simulink model "LQ_with_noise_realistic"  (R2023a)
settings: Solver=ode4  StartTime=0.0  StopTime=10  FixedStep=0.001  RelTol=1e-3
InitFcn:
  | Init_control;
values from neighbouring files (symbols this model uses):
  D = zeros(2,4)    [Init_control.m]
  klq = lqrd(A,B,Q,Rlq,Ts)    [Init_control.m]
  ModelInit_AngEuler = [0.4, 0.2, 0]    [Init_control.m]
  ModelInit_PosE = [0, 0, -100]    [Init_control.m]
  ModelInit_Rads = 557.142    [Init_control.m]
  ModelInit_RateB = [0, 0, 0]    [Init_control.m]
  ModelInit_VelB = [0, 0, 0]    [Init_control.m]
  P = [0.5 0 0 0 ... (first row only)    [Init_control.m]
  R = sqrt(2)/2*[-1 1 ... (first row only)    [Init_control.m]
  Ts = 0.002    [Init_control.m]
undefined symbols (not defined in the file or in its folder): ModelParam_envGravityAcc, ModelParam_motorCr, ModelParam_motorJm, ModelParam_motorT, ModelParam_motorWb, ModelParam_rotorCm, ModelParam_rotorCt, ModelParam_uavCCm, ModelParam_uavCd, ModelParam_uavJ, ModelParam_uavMass, ModelParam_uavR
libraries: simulink x4, sharedutil x2
settings Model: Creator=wsh  LastModifiedBy=matte
settings SolverCC: AlgebraicLoopSolver=TrustRegion
settings DataIOCC: ReturnWorkspaceOutputs=off
settings DebuggingCC: UnconnectedInputMsg=warning  UnconnectedOutputMsg=warning  UnconnectedLineMsg=warning  BusObjectLabelMismatch=error  ArithmeticOperatorsInVariantConditions=warning
settings ModelReferenceCC: EnableRefExpFcnMdlSchedulingChecks=on
settings SFSimCC: SimUseLocalCustomCode=off  CustomCodeUndefinedFunction=UseInterfaceOnly
settings RTWCC: RTWUseLocalCustomCode=off
settings CodeAppCC: StateflowObjectComments=on

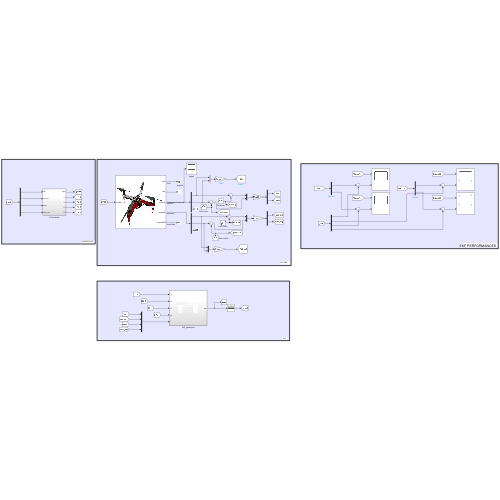
[thumbnail: Simulink's stored preview of the top-level diagram]
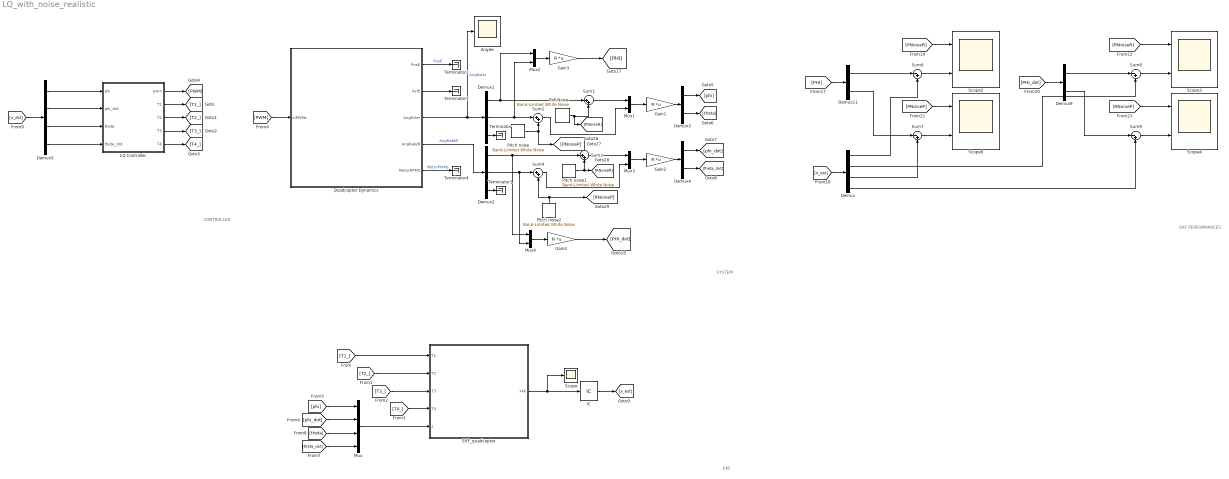
== system LQ_with_noise_realistic ==
  note: SYSTEM
  note: EKF
  note: CONTROLLER
  note: EKF PERFORMANCES
  Angles : Scope
  Demux : Demux
  Demux1 : Demux  Outputs=3
  Demux{3..4,9,11} (4 alike) : Demux  Outputs=2
  Demux2 : Demux  Outputs=3
  Demux5 : Demux
  EKF_quadcopter : Subsystem
  Gain{1..4} (4 alike) : Gain  Gain=R  Multiplication=Matrix(K*u) (u vector)
  IC : InitialCondition  Value=[0;0;0;0]
  LQ Controller : Subsystem
  Mux : Mux
  Mux{1..4} (4 alike) : Mux  Inputs=2
  Pitch noise : simulink/Sources/Band-Limited White Noise  Cov=[1.809123162388460e-08]  Ts=Ts  seed=[23341]
  Pitch noise1 : simulink/Sources/Band-Limited White Noise  Cov=[2.7827391e-06]  Ts=Ts  seed=[23341]
  Pitch noise2 : simulink/Sources/Band-Limited White Noise  Cov=[2.718240466492716e-06]  Ts=Ts  seed=[23341]
  Quadcopter Dynamics : Subsystem
      mask Display: image('./icon/F450.png');
  Roll Noise : simulink/Sources/Band-Limited White Noise  Cov=[1.936548166270313e-08]  Ts=Ts  seed=[23341]
  Scope : Scope
  Scope{2..4,6} (4 alike) : Scope  NumInputPorts=2
  Sum{1..4} (4 alike) : Sum  Inputs=|++
  Sum{6..9} (4 alike) : Sum  Inputs=|-+
  Terminator{,1..4} (5 alike) : Terminator
  wires:
  [x_est] -> Demux5/1
  [PWM] -> Quadcopter Dynamics/1(inPWMs)
  Demux4/2 -> [theta_dot]
  [phi] -> Mux/1
  [theta_dot] -> Mux/4
  Demux5/2 -> LQ Controller/2(phi_dot)
  Demux5/4 -> LQ Controller/4(theta_dot)
  Pitch noise/1 -> [PNoiseP], Sum2/2
  [T4_] -> EKF_quadcopter/4(T4)
  Sum4/1 -> Mux3/2
  IC/1 -> [x_est]
  LQ Controller/3(T2) -> [T2_]
  [theta] -> Mux/3
  Mux1/1 -> Gain1/1
  Demux2/1 -> Mux4/1, Sum3/1
  Sum2/1 -> Mux1/2
  EKF_quadcopter/1(xkk) -> IC/1, Scope/1
  LQ Controller/1(pwm) -> [PWM]
  LQ Controller/4(T3) -> [T3_]
  Demux5/3 -> LQ Controller/3(theta)
  [phi_dot] -> Mux/2
  Sum3/1 -> Mux3/1
  [T3_] -> EKF_quadcopter/3(T3)
  Pitch noise2/1 -> [RNoiseP], Sum4/2
  Demux2/2 -> Mux4/2, Sum4/1
  Demux3/1 -> [phi]
  LQ Controller/2(T1) -> [T1_]
  [T2_] -> EKF_quadcopter/2(T2)
  Quadcopter Dynamics/2(VelE) -> Terminator3/1
  Demux1/2 -> Mux2/2, Sum2/1
  LQ Controller/5(T4) -> [T4_]
  Gain1/1 -> Demux3/1
  Gain2/1 -> Demux4/1
  Roll Noise/1 -> [PNoiseR], Sum1/2
  Quadcopter Dynamics/1(PosE) -> Terminator2/1  "PosE"
  [T1_] -> EKF_quadcopter/1(T1)
  Demux3/2 -> [theta]
  Demux2/3 -> Terminator1/1
  Quadcopter Dynamics/5(MotorRPMS) -> Terminator4/1  "MotorPWMs"
  Demux1/3 -> Terminator/1
  Mux/1 -> EKF_quadcopter/5(z)
  Demux4/1 -> [phi_dot]
  Demux1/1 -> Mux2/1, Sum1/1
  Quadcopter Dynamics/4(AngRateB) -> Demux2/1  "AngRateB"
  Sum1/1 -> Mux1/1
  Demux5/1 -> LQ Controller/1(phi)
  Mux3/1 -> Gain2/1
  Demux/4 -> Sum9/2
  [PHI_dot] -> Demux9/1
  Demux9/1 -> Sum8/1
  Demux9/2 -> Sum9/1
  Demux11/2 -> Sum7/1
  Sum7/1 -> Scope6/2
  Demux/1 -> Sum6/2
  [PHI] -> Demux11/1
  Sum6/1 -> Scope2/2
  Demux11/1 -> Sum6/1
  Demux/3 -> Sum7/2
  Sum8/1 -> Scope3/2
  Sum9/1 -> Scope4/2
  Quadcopter Dynamics/3(AngEuler) -> Demux1/1, Angles/1  "AngEular"
  [x_est] -> Demux/1
  Demux/2 -> Sum8/2
  Pitch noise1/1 -> [RNoiseR], Sum3/2
  [PNoiseR] -> Scope2/1
  [PNoiseP] -> Scope6/1
  [RNoiseR] -> Scope3/1
  [RNoiseP] -> Scope4/1
  Mux2/1 -> Gain3/1
  Gain3/1 -> [PHI]
  Mux4/1 -> Gain4/1
  Gain4/1 -> [PHI_dot]

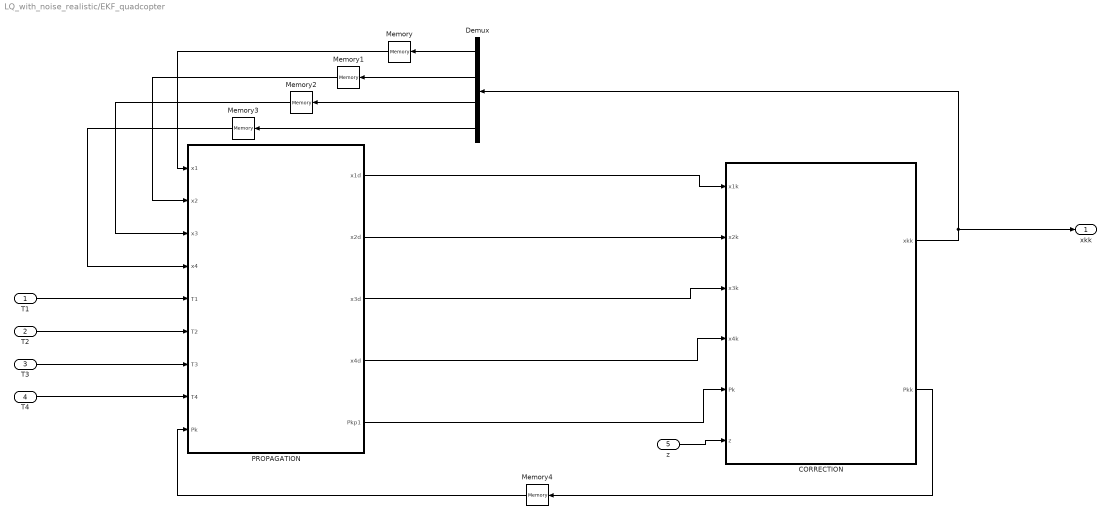
== system LQ_with_noise_realistic/EKF_quadcopter ==
  T1 : Inport
  T2 : Inport  Port=2
  T3 : Inport  Port=3
  T4 : Inport  Port=4
  z : Inport  Port=5
  CORRECTION : MATLAB Function  TreatAsAtomicUnit=on
  Demux : Demux
  Memory{,1..3} (4 alike) : Memory
  Memory4 : Memory  InitialCondition=P
  PROPAGATION : MATLAB Function  TreatAsAtomicUnit=on
  xkk : Outport
  wires:
  PROPAGATION/1(x1d) -> CORRECTION/1(x1k)
  PROPAGATION/2(x2d) -> CORRECTION/2(x2k)
  PROPAGATION/3(x3d) -> CORRECTION/3(x3k)
  PROPAGATION/4(x4d) -> CORRECTION/4(x4k)
  Memory4/1 -> PROPAGATION/9(Pk)
  T1/1 -> PROPAGATION/5(T1)
  T2/1 -> PROPAGATION/6(T2)
  T3/1 -> PROPAGATION/7(T3)
  T4/1 -> PROPAGATION/8(T4)
  PROPAGATION/5(Pkp1) -> CORRECTION/5(Pk)
  CORRECTION/2(Pkk) -> Memory4/1
  z/1 -> CORRECTION/6(z)
  Demux/1 -> Memory/1
  Demux/2 -> Memory1/1
  Demux/3 -> Memory2/1
  Demux/4 -> Memory3/1
  CORRECTION/1(xkk) -> Demux/1, xkk/1
  Memory/1 -> PROPAGATION/1(x1)
  Memory1/1 -> PROPAGATION/2(x2)
  Memory2/1 -> PROPAGATION/3(x3)
  Memory3/1 -> PROPAGATION/4(x4)

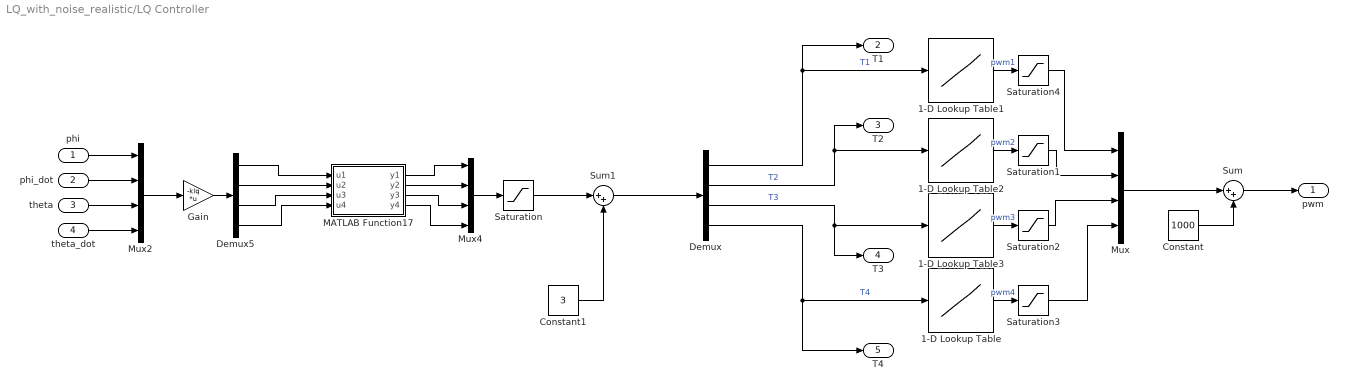
== system LQ_with_noise_realistic/LQ Controller ==
  phi : Inport
  phi_dot : Inport  Port=2
  theta : Inport  Port=3
  theta_dot : Inport  Port=4
  1-D Lookup Table : Lookup_n-D  NumberOfTableDimensions=1  BreakpointsForDimension1=[0;0.06477642396;0.16;0.63;2.44;4.43;6.92;8.77;10.52;11.63;12.03;12.09;12.091;12.092;12.093;12.094;12.095;12.096;12.097;12.098;12.099]  Table=[0;50;100;150;200;250;300;350;400;450;500;550;600;650;700;750;800;850;900;950;1000]  InternalRulePriority=Speed  RndMeth=Simplest
  1-D Lookup Table1 : Lookup_n-D  NumberOfTableDimensions=1  BreakpointsForDimension1=[0;0.02;0.06;0.29;0.73;1.07;1.88;2.91;4;5.06;6.71;7.86;9.41;10.86;11.45;11.82;12.07;12.31;12.52;12.74;12.75]  Table=[0;50;100;150;200;250;300;350;400;450;500;550;600;650;700;750;800;850;900;950;1000]  InternalRulePriority=Speed  RndMeth=Simplest
  1-D Lookup Table2 : Lookup_n-D  NumberOfTableDimensions=1  BreakpointsForDimension1=[0;0.05;0.39;1.67;3.19;5.57;8.07;10.01;10.71;11.06;11.42;11.53;11.55;11.551;11.552;11.553;11.554;11.555;11.556;11.557;11.558]  Table=[0;50;100;150;200;250;300;350;400;450;500;550;600;650;700;750;800;850;900;950;1000]  InternalRulePriority=Speed  RndMeth=Simplest
  1-D Lookup Table3 : Lookup_n-D  NumberOfTableDimensions=1  BreakpointsForDimension1=[0;0.06;0.23;0.89;2.47;3.9;5.86;7.81;9.42;10.12;10.6;11.01;11.34;11.39;11.391;11.392;11.393;11.394;11.395;11.396;11.397]  Table=[0;50;100;150;200;250;300;350;400;450;500;550;600;650;700;750;800;850;900;950;1000]  InternalRulePriority=Speed  RndMeth=Simplest
  Constant : Constant  Value=1000
  Constant1 : Constant  Value=3
  Demux : Demux
  Demux5 : Demux
  Gain : Gain  Gain=-klq  Multiplication=Matrix(K*u) (u vector)
  MATLAB Function17 : MATLAB Function  TreatAsAtomicUnit=on
  Mux : Mux
  Mux2 : Mux
  Mux4 : Mux
  Saturation : Saturate  UpperLimit=10  LowerLimit=0
  Saturation{1..4} (4 alike) : Saturate  UpperLimit=1000  LowerLimit=0
  Sum : Sum  Inputs=|++
  Sum1 : Sum  Inputs=|++
  pwm : Outport
  T1 : Outport  Port=2
  T2 : Outport  Port=3
  T3 : Outport  Port=4
  T4 : Outport  Port=5
  wires:
  Mux4/1 -> Saturation/1
  Mux2/1 -> Gain/1
  theta/1 -> Mux2/3
  1-D Lookup Table1/1 -> Saturation4/1  "pwm1"
  Saturation/1 -> Sum1/1
  Constant1/1 -> Sum1/2
  phi/1 -> Mux2/1
  1-D Lookup Table/1 -> Saturation3/1  "pwm4"
  Saturation4/1 -> Mux/1
  Demux5/2 -> MATLAB Function17/2(u2)
  Demux/1 -> T1/1, 1-D Lookup Table1/1  "T1"
  Gain/1 -> Demux5/1
  Saturation2/1 -> Mux/3
  Demux/4 -> T4/1, 1-D Lookup Table/1  "T4"
  Demux/3 -> T3/1, 1-D Lookup Table3/1  "T3"
  Demux5/4 -> MATLAB Function17/4(u4)
  Saturation1/1 -> Mux/2
  1-D Lookup Table3/1 -> Saturation2/1  "pwm3"
  Demux/2 -> 1-D Lookup Table2/1, T2/1  "T2"
  Sum1/1 -> Demux/1
  1-D Lookup Table2/1 -> Saturation1/1  "pwm2"
  MATLAB Function17/2(y2) -> Mux4/2
  Saturation3/1 -> Mux/4
  Demux5/3 -> MATLAB Function17/3(u3)
  MATLAB Function17/3(y3) -> Mux4/3
  MATLAB Function17/1(y1) -> Mux4/1
  MATLAB Function17/4(y4) -> Mux4/4
  Demux5/1 -> MATLAB Function17/1(u1)
  phi_dot/1 -> Mux2/2
  theta_dot/1 -> Mux2/4
  Sum/1 -> pwm/1
  Mux/1 -> Sum/1
  Constant/1 -> Sum/2

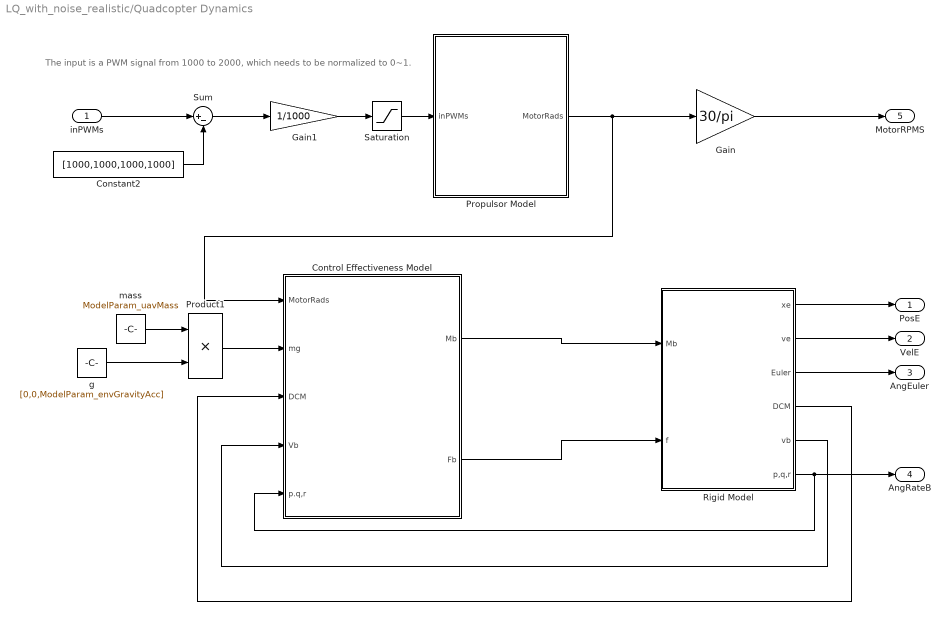
== system LQ_with_noise_realistic/Quadcopter Dynamics ==
  note: The input is a PWM signal from 1000 to 2000,
      | which needs to be normalized to 0~1.
  inPWMs : Inport
  Constant2 : Constant  Value=[1000,1000,1000,1000]
  Control Effectiveness Model : Subsystem
  Gain : Gain  Gain=30/pi
  Gain1 : Gain  Gain=1/1000
  Product1 : Product
  Propulsor Model : Subsystem
  Rigid Model : Subsystem
  Saturation : Saturate  UpperLimit=1  LowerLimit=0
  Sum : Sum  Inputs=|+-
  g : Constant  Value=[0,0,ModelParam_envGravityAcc]
  mass : Constant  Value=ModelParam_uavMass
  PosE : Outport  VectorParamsAs1DForOutWhenUnconnected=off
  VelE : Outport  Port=2  VectorParamsAs1DForOutWhenUnconnected=off
  AngEuler : Outport  Port=3  VectorParamsAs1DForOutWhenUnconnected=off
  AngRateB : Outport  Port=4  VectorParamsAs1DForOutWhenUnconnected=off
  MotorRPMS : Outport  Port=5  VectorParamsAs1DForOutWhenUnconnected=off
  wires:
  Saturation/1 -> Propulsor Model/1(inPWMs)
  Rigid Model/6("p,q,r ") -> Control Effectiveness Model/5(p.q,r), AngRateB/1
  mass/1 -> Product1/1
  Rigid Model/4(DCM) -> Control Effectiveness Model/3(DCM)
  Propulsor Model/1(MotorRads) -> Gain/1, Control Effectiveness Model/1(MotorRads)
  Gain1/1 -> Saturation/1
  Rigid Model/2(ve) -> VelE/1
  Sum/1 -> Gain1/1
  Product1/1 -> Control Effectiveness Model/2(mg)
  Rigid Model/5("vb ") -> Control Effectiveness Model/4(Vb)
  Rigid Model/1("xe ") -> PosE/1
  Rigid Model/3(Euler) -> AngEuler/1
  Control Effectiveness Model/1(Mb) -> Rigid Model/1(Mb)
  inPWMs/1 -> Sum/1
  Control Effectiveness Model/2(Fb) -> Rigid Model/2(f)
  Constant2/1 -> Sum/2
  g/1 -> Product1/2
  Gain/1 -> MotorRPMS/1

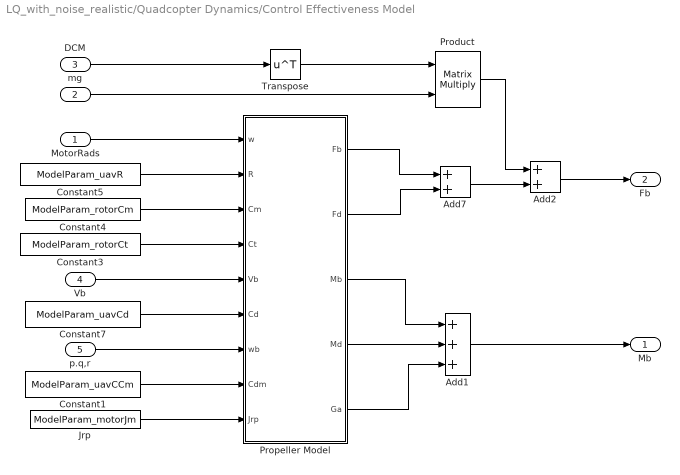
== system LQ_with_noise_realistic/Quadcopter Dynamics/Control Effectiveness Model ==
  MotorRads : Inport
  mg : Inport  Port=2
  DCM : Inport  Port=3
  Vb : Inport  Port=4
  p.q,r : Inport  Port=5
  Add1 : Sum  Inputs=+++
  Add2 : Sum
  Add7 : Sum
  Constant1 : Constant  Value=ModelParam_uavCCm
  Constant3 : Constant  Value=ModelParam_rotorCt
  Constant4 : Constant  Value=ModelParam_rotorCm
  Constant5 : Constant  Value=ModelParam_uavR
  Constant7 : Constant  Value=ModelParam_uavCd
  Jrp : Constant  Value=ModelParam_motorJm
  Product : Product  Multiplication=Matrix(*)
  Propeller Model : MATLAB Function  TreatAsAtomicUnit=on
  Transpose : Math  Operator=transpose  SignedPower=on
  Mb : Outport  VectorParamsAs1DForOutWhenUnconnected=off
  Fb : Outport  Port=2  VectorParamsAs1DForOutWhenUnconnected=off
  wires:
  Add2/1 -> Fb/1
  Constant3/1 -> Propeller Model/4(Ct)
  Propeller Model/2(Fd) -> Add7/2
  Add7/1 -> Add2/2
  Propeller Model/1(Fb) -> Add7/1
  Product/1 -> Add2/1
  mg/1 -> Product/2
  DCM/1 -> Transpose/1
  Constant7/1 -> Propeller Model/6(Cd)
  Vb/1 -> Propeller Model/5(Vb)
  Constant5/1 -> Propeller Model/2(R)
  Constant4/1 -> Propeller Model/3(Cm)
  MotorRads/1 -> Propeller Model/1(w)
  Transpose/1 -> Product/1
  Propeller Model/3(Mb) -> Add1/1
  Propeller Model/4(Md) -> Add1/2
  Add1/1 -> Mb/1
  p.q,r/1 -> Propeller Model/7(wb)
  Constant1/1 -> Propeller Model/8(Cdm)
  Jrp/1 -> Propeller Model/9(Jrp)
  Propeller Model/5(Ga) -> Add1/3

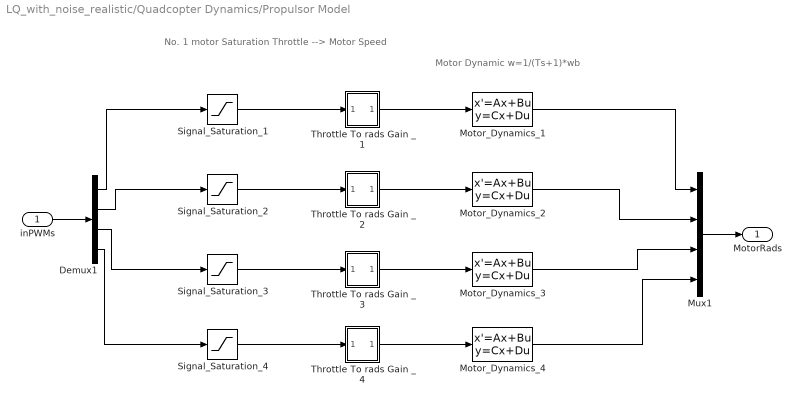
== system LQ_with_noise_realistic/Quadcopter Dynamics/Propulsor Model ==
  note: Motor Dynamic
      | w=1/(Ts+1)*wb
  note: No. 1 motor
      |
      |          Saturation             Throttle --> Motor Speed
  inPWMs : Inport
  Demux1 : Demux
  Motor_Dynamics_{1..4} (4 alike) : StateSpace  A=-1/ModelParam_motorT  C=1/ModelParam_motorT  D=0  InitialCondition=ModelInit_Rads*ModelParam_motorT
  Mux1 : Mux
  Signal_Saturation_{1..4} (4 alike) : Saturate  UpperLimit=1  LowerLimit=0
  Throttle To rads Gain _1 : Subsystem
  Throttle To rads Gain _2 : Subsystem
  Throttle To rads Gain _3 : Subsystem
  Throttle To rads Gain _4 : Subsystem
  MotorRads : Outport  VectorParamsAs1DForOutWhenUnconnected=off
  wires:
  Throttle To rads Gain _4/1(Out5) -> Motor_Dynamics_4/1
  Signal_Saturation_4/1 -> Throttle To rads Gain _4/1(In5)
  Signal_Saturation_3/1 -> Throttle To rads Gain _3/1(In5)
  Signal_Saturation_2/1 -> Throttle To rads Gain _2/1(In5)
  Motor_Dynamics_4/1 -> Mux1/4
  Motor_Dynamics_3/1 -> Mux1/3
  Motor_Dynamics_2/1 -> Mux1/2
  Motor_Dynamics_1/1 -> Mux1/1
  Signal_Saturation_1/1 -> Throttle To rads Gain _1/1(In5)
  Mux1/1 -> MotorRads/1
  Throttle To rads Gain _3/1(Out5) -> Motor_Dynamics_3/1
  Throttle To rads Gain _2/1(Out5) -> Motor_Dynamics_2/1
  Throttle To rads Gain _1/1(Out5) -> Motor_Dynamics_1/1
  inPWMs/1 -> Demux1/1
  Demux1/4 -> Signal_Saturation_4/1
  Demux1/3 -> Signal_Saturation_3/1
  Demux1/2 -> Signal_Saturation_2/1
  Demux1/1 -> Signal_Saturation_1/1

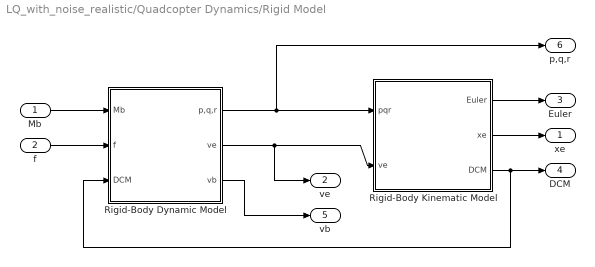
== system LQ_with_noise_realistic/Quadcopter Dynamics/Rigid Model ==
  Mb : Inport
  f : Inport  Port=2
  Rigid-Body Dynamic Model : Subsystem
  "Rigid-Body Kinematic Model " : Subsystem
  "xe " : Outport  VectorParamsAs1DForOutWhenUnconnected=off
  ve : Outport  Port=2  VectorParamsAs1DForOutWhenUnconnected=off
  Euler : Outport  Port=3  VectorParamsAs1DForOutWhenUnconnected=off
  DCM : Outport  Port=4  VectorParamsAs1DForOutWhenUnconnected=off
  "vb " : Outport  Port=5  VectorParamsAs1DForOutWhenUnconnected=off
  "p,q,r " : Outport  Port=6  VectorParamsAs1DForOutWhenUnconnected=off
  wires:
  Rigid-Body Dynamic Model/1("p,q,r ") -> "Rigid-Body Kinematic Model "/1(pqr), "p,q,r "/1
  "Rigid-Body Kinematic Model "/1(Euler) -> Euler/1
  "Rigid-Body Kinematic Model "/3(DCM) -> Rigid-Body Dynamic Model/3(DCM), DCM/1
  Mb/1 -> Rigid-Body Dynamic Model/1(Mb)
  f/1 -> Rigid-Body Dynamic Model/2(f)
  Rigid-Body Dynamic Model/2(ve) -> "Rigid-Body Kinematic Model "/2(ve), ve/1
  Rigid-Body Dynamic Model/3("vb ") -> "vb "/1
  "Rigid-Body Kinematic Model "/2("xe ") -> "xe "/1

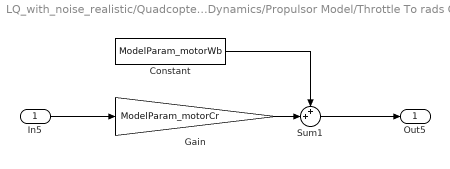
== system LQ_with_noise_realistic/Quadcopter Dynamics/Propulsor Model/Throttle To rads Gain _1 ==
  In5 : Inport
  Constant : Constant  Value=ModelParam_motorWb
  Gain : Gain  Gain=ModelParam_motorCr
  Sum1 : Sum  Inputs=++|
  Out5 : Outport  VectorParamsAs1DForOutWhenUnconnected=off
  wires:
  Constant/1 -> Sum1/1
  Gain/1 -> Sum1/2
  In5/1 -> Gain/1
  Sum1/1 -> Out5/1

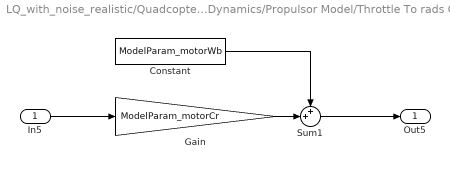
== system LQ_with_noise_realistic/Quadcopter Dynamics/Propulsor Model/Throttle To rads Gain _2 ==
  In5 : Inport
  Constant : Constant  Value=ModelParam_motorWb
  Gain : Gain  Gain=ModelParam_motorCr
  Sum1 : Sum  Inputs=++|
  Out5 : Outport  VectorParamsAs1DForOutWhenUnconnected=off
  wires:
  Sum1/1 -> Out5/1
  In5/1 -> Gain/1
  Gain/1 -> Sum1/2
  Constant/1 -> Sum1/1

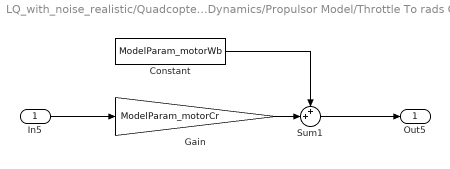
== system LQ_with_noise_realistic/Quadcopter Dynamics/Propulsor Model/Throttle To rads Gain _3 ==
  In5 : Inport
  Constant : Constant  Value=ModelParam_motorWb
  Gain : Gain  Gain=ModelParam_motorCr
  Sum1 : Sum  Inputs=++|
  Out5 : Outport  VectorParamsAs1DForOutWhenUnconnected=off
  wires:
  Constant/1 -> Sum1/1
  Gain/1 -> Sum1/2
  In5/1 -> Gain/1
  Sum1/1 -> Out5/1

== system LQ_with_noise_realistic/Quadcopter Dynamics/Propulsor Model/Throttle To rads Gain _4 ==
  In5 : Inport
  Constant : Constant  Value=ModelParam_motorWb
  Gain : Gain  Gain=ModelParam_motorCr
  Sum1 : Sum  Inputs=++|
  Out5 : Outport  VectorParamsAs1DForOutWhenUnconnected=off
  wires:
  Sum1/1 -> Out5/1
  In5/1 -> Gain/1
  Gain/1 -> Sum1/2
  Constant/1 -> Sum1/1

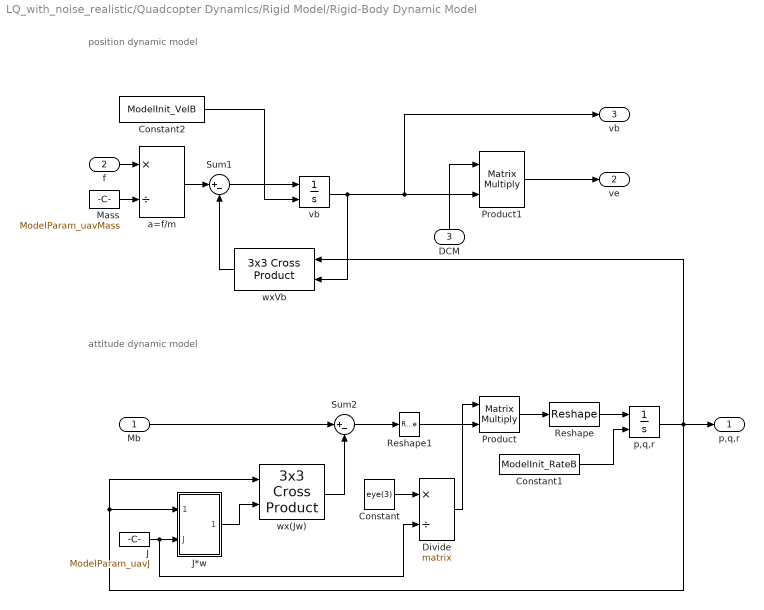
== system LQ_with_noise_realistic/Quadcopter Dynamics/Rigid Model/Rigid-Body Dynamic Model ==
  note: attitude dynamic model
  note: position dynamic model
  Mb : Inport
  f : Inport  Port=2
  DCM : Inport  Port=3
  " Mass " : Constant  Value=ModelParam_uavMass
  Constant : Constant  Value=eye(3)
  Constant1 : Constant  Value=ModelInit_RateB
  Constant2 : Constant  Value=ModelInit_VelB
  Divide : Product  Inputs=*/  Multiplication=Matrix(*)
  "J " : Constant  Value=ModelParam_uavJ
  J*w : Subsystem
  Product : Product  Multiplication=Matrix(*)
  Product1 : Product  Multiplication=Matrix(*)
  Reshape : Reshape  OutputDimensionality=Customize  OutputDimensions=[3,1]
  Reshape1 : Reshape  OutputDimensionality=Column vector (2-D)
  Sum1 : Sum  Inputs=|+-
  Sum2 : Sum  Inputs=|+-
  a=f/m : Product  Inputs=*/
  p,q,r : Integrator  InitialConditionSource=external
  vb : Integrator  InitialConditionSource=external
  wx(Jw) : sharedutil/3x3 Cross Product  aMode=aMode
  wxVb : sharedutil/3x3 Cross Product  aMode=aMode
  "p,q,r " : Outport  VectorParamsAs1DForOutWhenUnconnected=off
  ve : Outport  Port=2  VectorParamsAs1DForOutWhenUnconnected=off
  "vb " : Outport  Port=3  VectorParamsAs1DForOutWhenUnconnected=off
  wires:
  Product/1 -> Reshape/1
  Reshape1/1 -> Product/2
  Constant/1 -> Divide/1
  Divide/1 -> Product/1
  Sum2/1 -> Reshape1/1
  "J "/1 -> Divide/2, J*w/2(J)
  p,q,r/1 -> "p,q,r "/1, J*w/1(p q r), wx(Jw)/1, wxVb/1
  J*w/1("J*w ") -> wx(Jw)/2
  Mb/1 -> Sum2/1
  wx(Jw)/1 -> Sum2/2
  Constant2/1 -> vb/2
  f/1 -> a=f/m/1
  Product1/1 -> ve/1
  wxVb/1 -> Sum1/2
  a=f/m/1 -> Sum1/1
  Sum1/1 -> vb/1
  vb/1 -> Product1/2, "vb "/1, wxVb/2
  " Mass "/1 -> a=f/m/2
  DCM/1 -> Product1/1
  Reshape/1 -> p,q,r/1
  Constant1/1 -> p,q,r/2

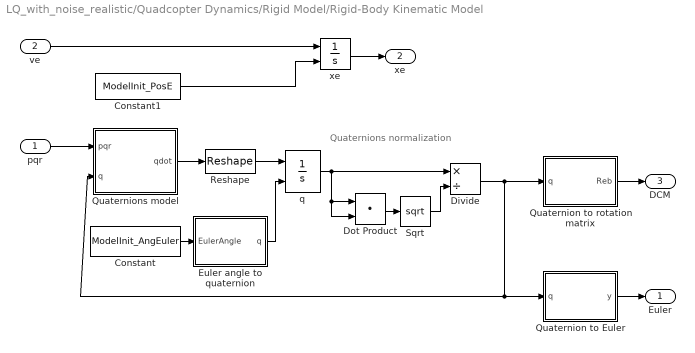
== system LQ_with_noise_realistic/Quadcopter Dynamics/Rigid Model/Rigid-Body Kinematic Model  ==
  note: Quaternions
      | normalization
  pqr : Inport
  ve : Inport  Port=2
  Constant : Constant  Value=ModelInit_AngEuler
  Constant1 : Constant  Value=ModelInit_PosE
  Divide : Product  Inputs=*/
  Dot Product : DotProduct  OutDataTypeStr=Inherit: Inherit via internal rule
  Euler angle to quaternion : MATLAB Function
  Quaternion to Euler : MATLAB Function
  Quaternion to rotation matrix : MATLAB Function
  Quaternions model : MATLAB Function  TreatAsAtomicUnit=on
  Reshape : Reshape  OutputDimensionality=Customize  OutputDimensions=[4,1]
  Sqrt : Sqrt
  q : Integrator  InitialConditionSource=external
  xe : Integrator  InitialConditionSource=external
  Euler : Outport  VectorParamsAs1DForOutWhenUnconnected=off
  "xe " : Outport  Port=2  VectorParamsAs1DForOutWhenUnconnected=off
  DCM : Outport  Port=3  VectorParamsAs1DForOutWhenUnconnected=off
  wires:
  Divide/1 -> Quaternion to rotation matrix/1(q), Quaternions model/2(q), Quaternion to Euler/1(q)
  Dot Product/1 -> Sqrt/1
  pqr/1 -> Quaternions model/1(pqr)
  q/1 -> Divide/1, Dot Product/1, Dot Product/2
  Quaternions model/1(qdot) -> Reshape/1
  Quaternion to rotation matrix/1(Reb) -> DCM/1
  Quaternion to Euler/1(y) -> Euler/1
  Constant/1 -> Euler angle to quaternion/1(EulerAngle)
  Euler angle to quaternion/1(q) -> q/2
  Reshape/1 -> q/1
  ve/1 -> xe/1
  xe/1 -> "xe "/1
  Constant1/1 -> xe/2
  Sqrt/1 -> Divide/2

== system LQ_with_noise_realistic/Quadcopter Dynamics/Rigid Model/Rigid-Body Dynamic Model/J*w ==
  p q r : Inport
  J : Inport  Port=2
  J*w : Product  Multiplication=Matrix(*)
  "J*w " : Outport  VectorParamsAs1DForOutWhenUnconnected=off
  wires:
  J*w/1 -> "J*w "/1
  J/1 -> J*w/1
  p q r/1 -> J*w/2

== matlab function LQ_with_noise_realistic/LQ Controller/MATLAB Function17 ==
  data: u1 input; y1 output; u2 input; u3 input; u4 input; y2 output; y3 output; y4 output
function [y1,y2,y3,y4] = fcn(u1,u2,u3,u4)

if u1 < 0
    u2 = u2 + abs(u1);
    u1 = u1+abs(u1);
end
if u2 < 0
    u2 = u2 + abs(u2);
    u1 = u1 + abs(u2);
end
if u3 < 0
    u3 = u3 + abs(u3);
    u4 = u4 + abs(u3);
end    
if u4 < 0
    u4 = u4 + abs(u4);
    u3 = u3 + abs(u4);
end
 y1 = u1;
 y2 = u2;
 y3 = u3;
 y4 = u4;

== matlab function LQ_with_noise_realistic/EKF_quadcopter/CORRECTION ==
  data: x1k input; xkk output; Pkk output; x2k input; x3k input; x4k input; Pk input; z input
function [xkk,Pkk] = fcn(x1k,x2k,x3k,x4k,Pk,z)

R = [1.936548166270313e-08 0 0 0;
     0 2.7827391e-06 0 0;
     0 0 1.809123162388460e-08 0;
     0 0 0 2.718240466492716e-06];

H = [1 0 0 0;
     0 1 0 0;
     0 0 1 0;
     0 0 0 1];

xk = [x1k;x2k;x3k;x4k];

y = z - H * xk;

K = Pk*(H')/(H*Pk*(H') + R);

xkk = xk + K * y;
Pkk = (eye(4)-K * H) * Pk;

== matlab function LQ_with_noise_realistic/EKF_quadcopter/PROPAGATION ==
  data: x1 input; x1d output; x2 input; x3 input; x4 input; T1 input; T2 input; T3 input; T4 input; x2d output; x3d output; x4d output; Pk input; Pkp1 output
function [x1d,x2d,x3d,x4d,Pkp1] = fcn(x1,x2,x3,x4,T1,T2,T3,T4,Pk)

m = 1.07;
L = 0.25;
d = 0.055;
J = 0.055;
g = 9.81;
Ts = 0.002;

Q = [1e-7 0 0 0;
     0 1e-4 0 0;
     0 0 1e-10 0;
     0 0 0 1e-7];

F11 = 0;
F12 = 1;
F13 = 0;
F14 = 0;

F21 = m*g*d/J*cos(x1)+T2*(-L*sin(x1)-d*cos(x1))/J-T1*(-L*sin(x1)+d*cos(x1))/J;
F22 = 0;
F23 = 0;
F24 = 0;

F31 = 0;
F32 = 0;
F33 = 0;
F34 = 1;


F41 = 0;
F42 = 0;
F43 = m*g*d*cos(x3)/J+T4*(-L*sin(x3)-d*cos(x3))/J-T3*(-L*sin(x3)+d*cos(x3))/J;
F44 = 0;

F = [F11 F12 F13 F14;
     F21 F22 F23 F24;
     F31 F32 F33 F34;
     F41 F42 F43 F44];

PHI = expm(F * Ts);

x1d_dot = x2;
x2d_dot = m*g*d*sin(x1)/J + T2*(L*cos(x1)-d*sin(x1))/J - T1*(L*cos(x1) + ...
    d*sin(x1))/J;
x3d_dot = x4;
x4d_dot = m*g*d*sin(x3)/J + T4*(L*cos(x3)-d*sin(x3))/J - T3*(L*cos(x3) + ...
    d*sin(x3))/J;

x1d = x1 + x1d_dot*Ts;
x2d = x2 + x2d_dot*Ts;
x3d = x3 + x3d_dot*Ts;
x4d = x4 + x4d_dot*Ts;

Pkp1 = PHI * Pk * (PHI') + Q;

== matlab function LQ_with_noise_realistic/Quadcopter Dynamics/Rigid Model/Rigid-Body Kinematic Model /Quaternion to rotation matrix ==
  data: q input; Reb output
function Reb = fcn(q)
%Function description;
%  The rotation matrix of the Aircraft-Body Coordinate Frame (ABCF) to the
%  Earth-Fixed Coordinate Frame (EFCF) is obtained from the quaternions
Reb = [q(1)*q(1) + q(2)*q(2) - q(3)*q(3) - q(4)*q(4), 2*(q(2)*q(3) - q(1)*q(4)), 2*(q(2)*q(4) + q(1)*q(3))
           2*(q(2)*q(3) + q(1)*q(4)), q(1)*q(1) - q(2)*q(2) + q(3)*q(3) - q(4)*q(4), 2*(q(3)*q(4) - q(1)*q(2))
           2*(q(2)*q(4) - q(1)*q(3)), 2*(q(3)*q(4) + q(1)*q(2)), q(1)*q(1) - q(2)*q(2) - q(3)*q(3) + q(4)*q(4)];

== matlab function LQ_with_noise_realistic/Quadcopter Dynamics/Rigid Model/Rigid-Body Kinematic Model /Quaternion to Euler ==
  data: q input; y output
function y = fcn(q)
 %Function description:
%  Quaternions to Euler
phi = atan2(2*(q(1)*q(2) + q(3)*q(4)), (1 - 2*(q(2)*q(2) + q(3)*q(3))));
theta = asin(2*(q(1)*q(3) - q(2)*q(4)));
psi = atan2(2*(q(1)*q(4) + q(2)*q(3)), (1 - 2*(q(3)*q(3) + q(4)*q(4))));
y = [phi theta psi];

== matlab function LQ_with_noise_realistic/Quadcopter Dynamics/Rigid Model/Rigid-Body Kinematic Model /Quaternions model ==
  data: pqr input; qdot output; q input
function qdot = fcn(pqr, q)
%Function description:
%  Quaternions model
qdot = 0.5*[0, -pqr(1), -pqr(2), -pqr(3); pqr(1), 0, pqr(3), -pqr(2); pqr(2), -pqr(3), 0, pqr(1); pqr(3), pqr(2), -pqr(1), 0]*q;

== matlab function LQ_with_noise_realistic/Quadcopter Dynamics/Rigid Model/Rigid-Body Kinematic Model /Euler angle to quaternion ==
  data: EulerAngle input; q output
function q = fcn(EulerAngle)
%Function description:
%  Get quaternions from Euler angle
q0 =  cos(EulerAngle(1)/2)*cos(EulerAngle(2)/2)*cos(EulerAngle(3)/2) + sin(EulerAngle(1)/2)*sin((EulerAngle(2)/2))*sin((EulerAngle(3)/2));
q1 = sin(EulerAngle(1)/2)*cos(EulerAngle(2)/2)*cos(EulerAngle(3)/2) - cos(EulerAngle(1)/2)*sin((EulerAngle(2)/2))*sin((EulerAngle(3)/2));
q2 = cos(EulerAngle(1)/2)*sin(EulerAngle(2)/2)*cos(EulerAngle(3)/2) + sin(EulerAngle(1)/2)*cos((EulerAngle(2)/2))*sin((EulerAngle(3)/2));
q3 = cos(EulerAngle(1)/2)*cos(EulerAngle(2)/2)*sin(EulerAngle(3)/2) - sin(EulerAngle(1)/2)*sin((EulerAngle(2)/2))*cos((EulerAngle(3)/2));
q = [q0 q1 q2 q3]';

== matlab function LQ_with_noise_realistic/Quadcopter Dynamics/Control Effectiveness Model/Propeller Model ==
  data: w input; R input; Fb output; Fd output; Mb output; Cm input; Ct input; Vb input; Cd input; wb input; Md output; Cdm input; Jrp input; Ga output
function [Fb, Fd, Mb, Md, Ga] = fcn(w, R, Cm, Ct, Vb, Cd,wb, Cdm, Jrp)
 %Function description:
 %  Obtain the force and torque acting on the body. The airframe of the
 %  quadrotor is as follows:
 %3↓   1↑
 %  \ /
 %  / \
 %2↑   4↓
 %↑ stands for counterclockwise and ↓stands for clockwise.
 %Input：
 %  w: motor speed，unit：rad/s
 %  R: body radius(m)
 %  Cm: torque coefficient
 %  Ct: thrust coefficient
 %  Vb: aircraft speed in the body coordinate system
 %  Cd: damping coefficient
 %  wb: angular velocity in the body coordinate system
 %  Cdm: damping moment coefficient vector
 %  Jrp:  moment of inertia of motor rotor + propeller
 %Output:
 %  Fb: thrust under the body coordinate system
 %  Fd: aerodynamic force under the body coordinate system
 %  Mb: torque under the body coordinate system
 %  Md: aerodynamic moment
 %  Ga: gyro moment
 M_rctcm = [-sin(pi/4)*R*Ct, sin(pi/4)*R*Ct, sin(pi/4)*R*Ct, -sin(pi/4)*R*Ct;
            sin(pi/4)*R*Ct, -sin(pi/4)*R*Ct, sin(pi/4)*R*Ct, -sin(pi/4)*R*Ct;
            Cm, Cm, -Cm, -Cm];
 Mb = M_rctcm*(w.^2);  % torque
 
 Fb = [0; 0; -sum(Ct*(w.^2))];  % thrust
 Fd = -Cd*Vb.*abs(Vb)*0.5;  % aerodynamic force
 Md = -Cdm.*wb.*abs(wb);  % aerodynamic moment
 % gyro moment
 Ga = zeros(3,1);
 Ga(1) = Jrp*wb(2)*( w(1) + w(2) - w(3) - w(4));
 Ga(2) = Jrp*wb(1)*(-w(1) - w(2) + w(3) + w(4));
end
